simulink model "ADRConSiaAUV_ex02"  (R2021a)
settings: Solver=ode1  StartTime=0  StopTime=100  FixedStep=h  MaxStep=0.05  MinStep=0.005  RelTol=0.01
values from neighbouring files (symbols this model uses):
  b0 = 0.06    [tuning0325.m]
  h0 = 1.0    (= 1)    [tuning0325.m]
  kd = 10    [NPS_RBFNN01.m]    (also in SiaAUV_RBFNN01.m; SiaAUV_RBFNN02.m; SiaAUV_RBFNN03.m; tuning0325.m = 90)
  ki = 0.9    [tuning0325.m]
  kp = 6    [NPS_RBFNN01.m]    (also in SiaAUV_RBFNN01.m; SiaAUV_RBFNN02.m; SiaAUV_RBFNN03.m; tuning0325.m = 50)
  r0 = 0.8    [tuning0325.m]
  w0 = 80    [tuning0325.m]
  wc = 0.5    [tuning0325.m]
libraries: mssSimulink x12, simulink x3
settings Model: Creator=thor  LastModifiedBy=owenga
settings SolverCC: InitialStep=0.01  AlgebraicLoopSolver=TrustRegion  AutoInsertRateTranBlk=on
settings DataIOCC: LimitDataPoints=on  SaveFormat=Array  SignalLoggingSaveFormat=ModelDataLogs  ReturnWorkspaceOutputs=off  SignalLoggingName=sigsOut
settings OptimizationCC: BooleanDataType=off  InitFltsAndDblsToZero=on  LifeSpan=inf
settings DebuggingCC: SaveWithParameterizedLinksMsg=none  UnderspecifiedInitializationDetection=Classic  MergeDetectMultiDrivingBlocksExec=none  SignalResolutionControl=TryResolveAllWithWarning  MultiTaskDSMMsg=warning  MultiTaskCondExecSysMsg=none  FcnCallInpInsideContextMsg=warning  SFUnexpectedBacktrackingDiag=warning  SFNoUnconditionalDefaultTransitionDiag=warning  SFExecutionAtInitializationDiag=none  SFMachineParentedDataDiag=warning  ArithmeticOperatorsInVariantConditions=warning
settings HardwareCC: ProdBitPerPointer=32  ProdBitPerSizeT=32  ProdBitPerPtrDiffT=32  ProdLargestAtomicFloat=None  ProdIntDivRoundTo=Undefined  ProdEndianess=Unspecified  ProdWordSize=32  ProdHWDeviceType=32-bit Generic  TargetUnknown=on
settings ModelReferenceCC: PropagateSignalLabelsOutOfModel=off
settings CodeAppCC: StateflowObjectComments=on
settings GRTTargetCC: TargetFcnLib=ansi_tfl_tmw.mat  TargetLangStandard=C89/C90 (ANSI)  ModelReferenceCompliant=off  CombineOutputUpdateFcns=off  MatFileLogging=off  GRTInterface=on
settings ConfigComp: CovMetricSettings=dw  CovSaveCumulativeToWorkspaceVar=on  CovSaveSingleToWorkspaceVar=on

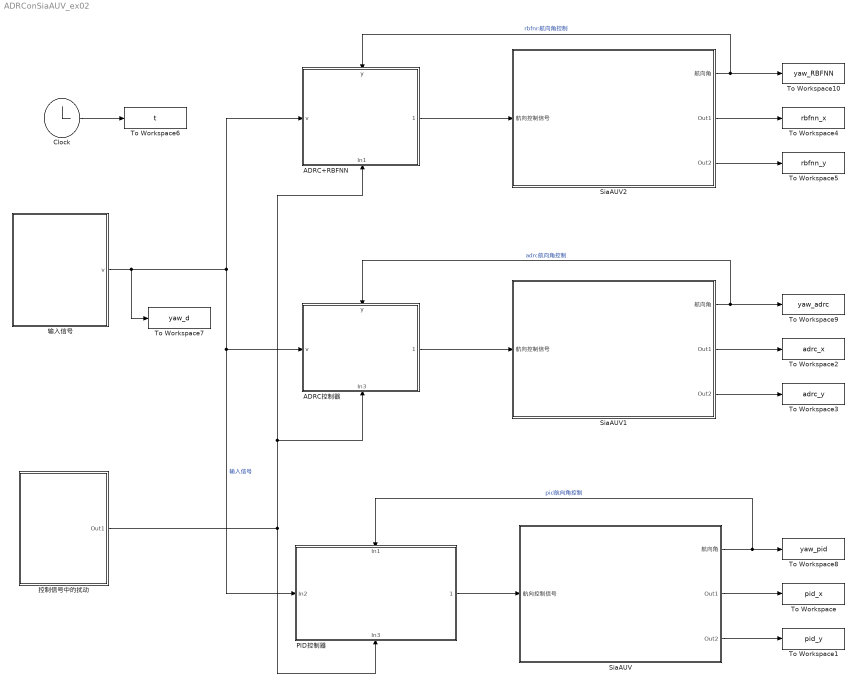
== system ADRConSiaAUV_ex02 ==
  ADRC+RBFNN : Subsystem
      settings: PortSchema="{\"entries\":[{\"content\":{\"sides\":[{\"content\":{\"connectorIds\":[\"In1\"]},\"type\":\"ConnectorPlacement.EquallySpacedRectSide\",\"uuid\":\"900b6237-364a-4e14-939f-8bb5c6ed2e80\"},{\"content\":{\"connectorIds\":[\"Out1\"],\"side\":\"RIGHT\"},\"type\":\"ConnectorPlacement.EquallySpacedRectSide\",\"uuid\":\"a73f2338-5f87-4ee3-a03f-e680a590baff\"},{\"content\":{\"connectorIds\":[\"In2\"],\"side\":\"TOP\"},\"type\":\"ConnectorPlacement.EquallySpacedRectSide\",\"uuid\":\"06c6f34a-b3b2-48d7-b766-545f9568804e\"},{\"content\":{\"connectorIds\":[\"In3\"],\"side\":\"BOTTOM\"},\"type\":\"ConnectorPlacement.EquallySpacedRectSide\",\"uuid\":\"dbaae600-9c02-41f2-84b1-a2698d1307a6\"}]},\"type\":\"ConnectorPlacement.EquallySpacedConnector\",\"uuid\":\"fa40750b-3e1f-406a-9fab-e6d49e04910d\"}],\"packageUris\":[\"http://schema.mathworks.com/mf0/Connector/R2020b\"],\"version\":\"1.0\"}"
  ADRC控制器 : Subsystem
      settings: PortSchema="{\"entries\":[{\"content\":{\"sides\":[{\"content\":{\"connectorIds\":[\"In1\"]},\"type\":\"ConnectorPlacement.EquallySpacedRectSide\",\"uuid\":\"32724ae5-2155-4067-bb70-245a7591a597\"},{\"content\":{\"connectorIds\":[\"Out1\"],\"side\":\"RIGHT\"},\"type\":\"ConnectorPlacement.EquallySpacedRectSide\",\"uuid\":\"c5581aa9-8b72-4f1c-be64-cbd035fc9c4e\"},{\"content\":{\"connectorIds\":[\"In2\"],\"side\":\"TOP\"},\"type\":\"ConnectorPlacement.EquallySpacedRectSide\",\"uuid\":\"d8180c3e-1afe-4e75-b9a0-261cdd740691\"},{\"content\":{\"connectorIds\":[\"In3\"],\"side\":\"BOTTOM\"},\"type\":\"ConnectorPlacement.EquallySpacedRectSide\",\"uuid\":\"8af971cc-81cd-4e66-97aa-994f656c03e7\"}]},\"type\":\"ConnectorPlacement.EquallySpacedConnector\",\"uuid\":\"6b6572c2-6358-4ebe-8c55-bca9fb0d42f3\"}],\"packageUris\":[\"http://schema.mathworks.com/mf0/Connector/R2020b\"],\"version\":\"1.0\"}"
  Clock : Clock
  PID控制器 : Subsystem
      settings: PortSchema="{\"entries\":[{\"content\":{\"sides\":[{\"content\":{\"connectorIds\":[\"In1\"]},\"type\":\"ConnectorPlacement.EquallySpacedRectSide\",\"uuid\":\"32724ae5-2155-4067-bb70-245a7591a597\"},{\"content\":{\"connectorIds\":[\"Out1\"],\"side\":\"RIGHT\"},\"type\":\"ConnectorPlacement.EquallySpacedRectSide\",\"uuid\":\"c5581aa9-8b72-4f1c-be64-cbd035fc9c4e\"},{\"content\":{\"connectorIds\":[\"In2\"],\"side\":\"TOP\"},\"type\":\"ConnectorPlacement.EquallySpacedRectSide\",\"uuid\":\"d8180c3e-1afe-4e75-b9a0-261cdd740691\"},{\"content\":{\"connectorIds\":[\"In3\"],\"side\":\"BOTTOM\"},\"type\":\"ConnectorPlacement.EquallySpacedRectSide\",\"uuid\":\"f6cb4f31-ad77-48c7-baef-a98beb6e51e5\"}]},\"type\":\"ConnectorPlacement.EquallySpacedConnector\",\"uuid\":\"6b6572c2-6358-4ebe-8c55-bca9fb0d42f3\"}],\"packageUris\":[\"http://schema.mathworks.com/mf0/Connector/R2020b\"],\"version\":\"1.0\"}"
  SiaAUV : Subsystem
  SiaAUV1 : Subsystem
  SiaAUV2 : Subsystem
  To Workspace : ToWorkspace  VariableName=pid_x  SampleTime=-1
  To Workspace1 : ToWorkspace  VariableName=pid_y  SampleTime=-1
  To Workspace10 : ToWorkspace  VariableName=yaw_RBFNN  SampleTime=-1
  To Workspace2 : ToWorkspace  VariableName=adrc_x  SampleTime=-1
  To Workspace3 : ToWorkspace  VariableName=adrc_y  SampleTime=-1
  To Workspace4 : ToWorkspace  VariableName=rbfnn_x  SampleTime=-1
  To Workspace5 : ToWorkspace  VariableName=rbfnn_y  SampleTime=-1
  To Workspace6 : ToWorkspace  VariableName=t  SampleTime=-1
  To Workspace7 : ToWorkspace  VariableName=yaw_d  SampleTime=-1
  To Workspace8 : ToWorkspace  VariableName=yaw_pid  SampleTime=-1
  To Workspace9 : ToWorkspace  VariableName=yaw_adrc  SampleTime=-1
  控制信号中的扰动 : Subsystem
  输入信号 : Subsystem
  wires:
  控制信号中的扰动/1(Out1) -> ADRC控制器/3(In3), ADRC+RBFNN/3(In1), PID控制器/3(In3)
  SiaAUV/1(航向角) -> PID控制器/2(In1), To Workspace8/1  "pid航向角控制"
  SiaAUV/2(Out1) -> To Workspace/1
  SiaAUV/3(Out2) -> To Workspace1/1
  输入信号/1(v) -> ADRC+RBFNN/1(v), PID控制器/1(In2), ADRC控制器/1(v), To Workspace7/1  "输入信号"
  ADRC控制器/1(1) -> SiaAUV1/1(航向控制信号)
  SiaAUV1/2(Out1) -> To Workspace2/1
  SiaAUV1/3(Out2) -> To Workspace3/1
  SiaAUV1/1(航向角) -> To Workspace9/1, ADRC控制器/2(y)  "adrc航向角控制"
  ADRC+RBFNN/1(1) -> SiaAUV2/1(航向控制信号)
  SiaAUV2/1(航向角) -> To Workspace10/1, ADRC+RBFNN/2(y)  "rbfnn航向角控制"
  SiaAUV2/2(Out1) -> To Workspace4/1
  SiaAUV2/3(Out2) -> To Workspace5/1
  PID控制器/1(1) -> SiaAUV/1(航向控制信号)
  Clock/1 -> To Workspace6/1

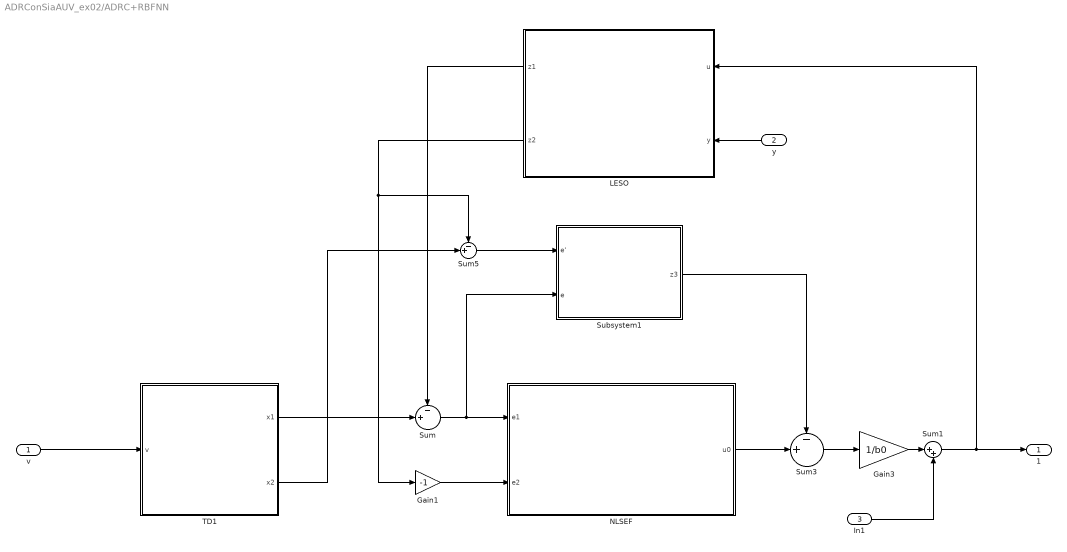
== system ADRConSiaAUV_ex02/ADRC+RBFNN ==
  v : Inport
  y : Inport  Port=2
  In1 : Inport  Port=3
  Gain1 : Gain  Gain=-1
  Gain3 : Gain  Gain=1/b0
  LESO : Subsystem
  NLSEF : Subsystem
  Subsystem1 : Subsystem
  Sum : Sum  Inputs=-+|
  Sum1 : Sum  Inputs=|++
  Sum3 : Sum  Inputs=-+|
  Sum5 : Sum  Inputs=-+|  SaturateOnIntegerOverflow=on
  TD1 : Subsystem
  1 : Outport
  wires:
  LESO/1(z1) -> Sum/1
  TD1/2(x2) -> Sum5/2
  NLSEF/1(u0) -> Sum3/2
  Sum5/1 -> Subsystem1/1(e')
  Sum3/1 -> Gain3/1
  Gain1/1 -> NLSEF/2(e2)
  y/1 -> LESO/2(y)
  Sum1/1 -> 1/1, LESO/1(u)
  LESO/2(z2) -> Gain1/1, Sum5/1
  Subsystem1/1(z3) -> Sum3/1
  Sum/1 -> Subsystem1/2(e), NLSEF/1(e1)
  Gain3/1 -> Sum1/1
  In1/1 -> Sum1/2
  v/1 -> TD1/1(v)
  TD1/1(x1) -> Sum/2

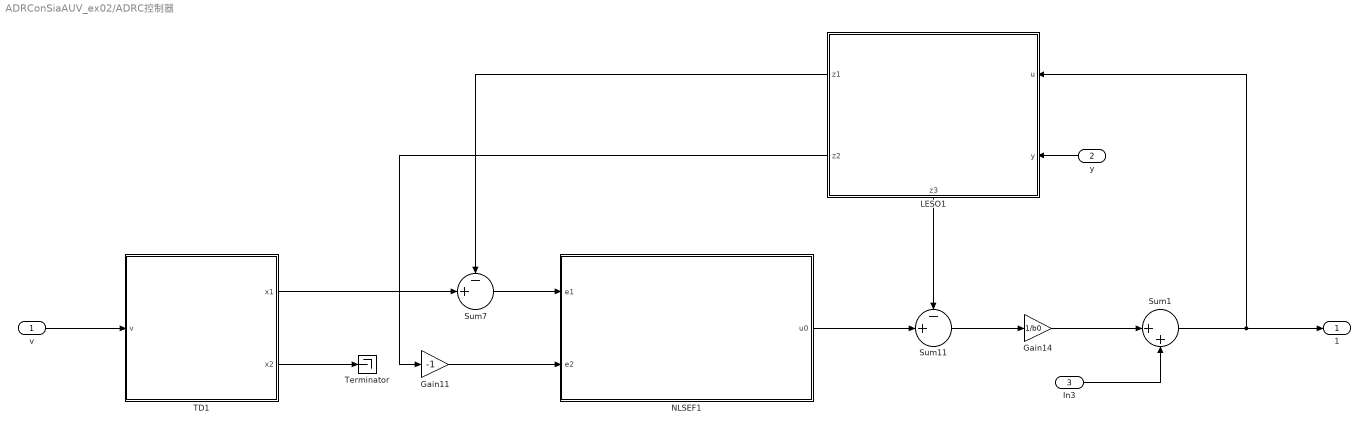
== system ADRConSiaAUV_ex02/ADRC控制器 ==
  v : Inport
  y : Inport  Port=2
  In3 : Inport  Port=3
  Gain11 : Gain  Gain=-1
  Gain14 : Gain  Gain=1/b0
  LESO1 : Subsystem
      settings: PortSchema="{\"entries\":[{\"content\":{\"sides\":[{\"content\":{\"connectorIds\":[\"In1\",\"In2\"]},\"type\":\"ConnectorPlacement.EquallySpacedRectSide\",\"uuid\":\"d43d14c0-31a6-421f-9c22-52af5a429c00\"},{\"content\":{\"connectorIds\":[\"Out1\",\"Out2\"],\"side\":\"RIGHT\"},\"type\":\"ConnectorPlacement.EquallySpacedRectSide\",\"uuid\":\"46ebe2a2-48dd-422a-a4e2-a7c2a0b0d12b\"},{\"content\":{\"connectorIds\":[],\"side\":\"TOP\"},\"type\":\"ConnectorPlacement.EquallySpacedRectSide\",\"uuid\":\"15fa3bf3-1107-4b09-8c97-c0a9c58ebc3c\"},{\"content\":{\"connectorIds\":[\"Out3\"],\"side\":\"BOTTOM\"},\"type\":\"ConnectorPlacement.EquallySpacedRectSide\",\"uuid\":\"1b52abbe-f0a6-429e-b5ef-1092e11e8dfa\"}]},\"type\":\"ConnectorPlacement.EquallySpacedConnector\",\"uuid\":\"aa00def6-f836-4863-9222-5c98f4f3fade\"}],\"packageUris\":[\"http://schema.mathworks.com/mf0/Connector/R2020b\"],\"version\":\"1.0\"}"
  NLSEF1 : Subsystem
  Sum1 : Sum  Inputs=|++
  Sum11 : Sum  Inputs=-+|
  Sum7 : Sum  Inputs=-+|
  TD1 : Subsystem
  Terminator : Terminator
  1 : Outport
  wires:
  LESO1/1(z1) -> Sum7/1
  Sum11/1 -> Gain14/1
  Gain11/1 -> NLSEF1/2(e2)
  TD1/1(x1) -> Sum7/2
  NLSEF1/1(u0) -> Sum11/2
  y/1 -> LESO1/2(y)
  Sum1/1 -> LESO1/1(u), 1/1
  TD1/2(x2) -> Terminator/1
  LESO1/2(z2) -> Gain11/1
  In3/1 -> Sum1/2
  Gain14/1 -> Sum1/1
  LESO1/3(z3) -> Sum11/1
  v/1 -> TD1/1(v)
  Sum7/1 -> NLSEF1/1(e1)

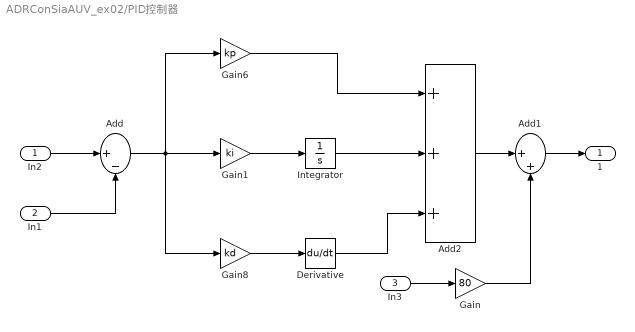
== system ADRConSiaAUV_ex02/PID控制器 ==
  In2 : Inport
  In1 : Inport  Port=2
  In3 : Inport  Port=3
  Add : Sum  Inputs=|+-
  Add1 : Sum  Inputs=|++
  Add2 : Sum  Inputs=+++
  Derivative : Derivative
  Gain : Gain  Gain=80
  Gain1 : Gain  Gain=ki
  Gain6 : Gain  Gain=kp
  Gain8 : Gain  Gain=kd
  Integrator : Integrator
  1 : Outport
  wires:
  In1/1 -> Add/2
  Add1/1 -> 1/1
  In2/1 -> Add/1
  In3/1 -> Gain/1
  Add2/1 -> Add1/1
  Derivative/1 -> Add2/3
  Gain8/1 -> Derivative/1
  Gain1/1 -> Integrator/1
  Integrator/1 -> Add2/2
  Gain6/1 -> Add2/1
  Add/1 -> Gain1/1, Gain8/1, Gain6/1
  Gain/1 -> Add1/2

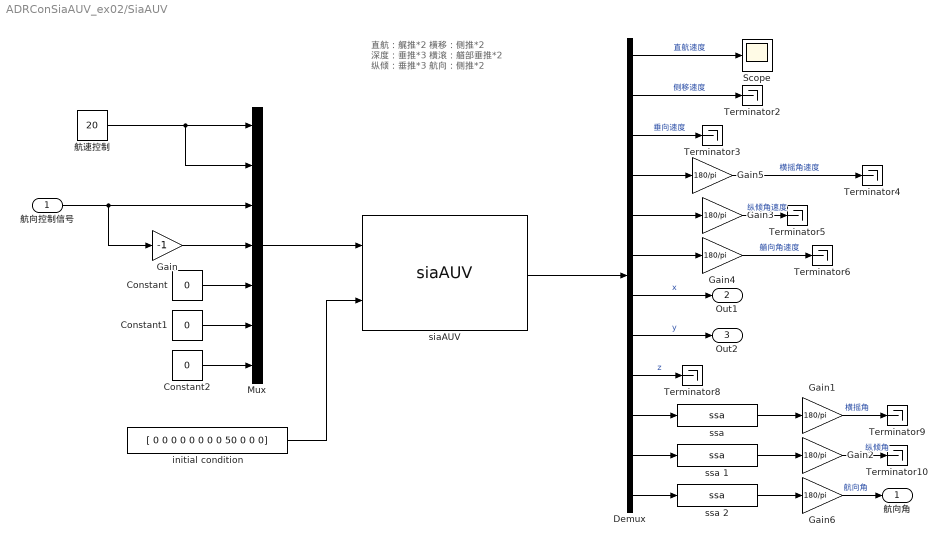
== system ADRConSiaAUV_ex02/SiaAUV ==
  note: 直航：艉推*2
      | 横移：侧推*2
      | 深度：垂推*3
      | 横滚：艏部垂推*2
      | 纵倾：垂推*3
      | 航向：侧推*2
  航向控制信号 : Inport
  Constant : Constant  Value=0
  Constant1 : Constant  Value=0
  Constant2 : Constant  Value=0
  Demux : Demux  Outputs=12
  Gain : Gain  Gain=-1
  Gain{1..6} (6 alike) : Gain  Gain=180/pi
  Mux : Mux  Inputs=[1 1 1 1 1 1 1]
  Scope : Scope
  Terminator{2..6,8..10} (8 alike) : Terminator
  initial condition : Constant  Value=[ 0 0 0 0 0 0 0 0 50 0 0 0]
  siaAUV : mssSimulink/Marine craft models/siaAUV  SystemSampleTime=-1  VariantActivationTime=update diagram  Latency=0  AutoFrameSizeCalculation=off
      settings: SourceProductName=Under Water Robot Toolbox
  "ssa " : mssSimulink/Utilities/Math Operations/ssa  SystemSampleTime=-1  VariantActivationTime=update diagram  Latency=0  AutoFrameSizeCalculation=off
      settings: SourceProductName=Under Water Robot Toolbox
  ssa 1 : mssSimulink/Utilities/Math Operations/ssa  SystemSampleTime=-1  VariantActivationTime=update diagram  Latency=0  AutoFrameSizeCalculation=off
      settings: SourceProductName=Under Water Robot Toolbox
  ssa 2 : mssSimulink/Utilities/Math Operations/ssa  SystemSampleTime=-1  VariantActivationTime=update diagram  Latency=0  AutoFrameSizeCalculation=off
      settings: SourceProductName=Under Water Robot Toolbox
  航速控制 : Constant  Value=20
  航向角 : Outport
  Out1 : Outport  Port=2
  Out2 : Outport  Port=3
  wires:
  Gain3/1 -> Terminator5/1  "纵倾角速度"
  Demux/3 -> Terminator3/1  "垂向速度"
  Gain1/1 -> Terminator9/1  "横摇角"
  Demux/4 -> Gain5/1
  Constant/1 -> Mux/5
  Gain/1 -> Mux/4
  Demux/12 -> ssa 2/1
  siaAUV/1 -> Demux/1
  ssa 1/1 -> Gain2/1
  Demux/5 -> Gain3/1
  Demux/9 -> Terminator8/1  "z"
  Demux/7 -> Out1/1  "x"
  Constant2/1 -> Mux/7
  ssa 2/1 -> Gain6/1
  Demux/1 -> Scope/1  "直航速度"
  Gain4/1 -> Terminator6/1  "艏向角速度"
  Demux/10 -> "ssa "/1
  Constant1/1 -> Mux/6
  initial condition/1 -> siaAUV/2
  "ssa "/1 -> Gain1/1
  Demux/6 -> Gain4/1
  Gain2/1 -> Terminator10/1  "纵倾角"
  Gain5/1 -> Terminator4/1  "横摇角速度"
  航速控制/1 -> Mux/2, Mux/1
  Demux/11 -> ssa 1/1
  Demux/2 -> Terminator2/1  "侧移速度"
  Gain6/1 -> 航向角/1  "航向角"
  Mux/1 -> siaAUV/1
  Demux/8 -> Out2/1  "y"
  航向控制信号/1 -> Gain/1, Mux/3

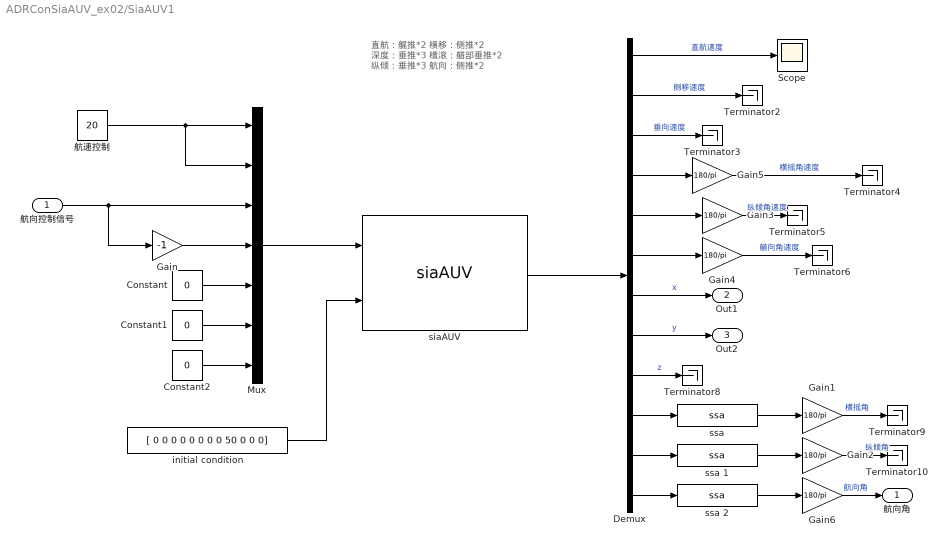
== system ADRConSiaAUV_ex02/SiaAUV1 ==
  note: 直航：艉推*2
      | 横移：侧推*2
      | 深度：垂推*3
      | 横滚：艏部垂推*2
      | 纵倾：垂推*3
      | 航向：侧推*2
  航向控制信号 : Inport
  Constant : Constant  Value=0
  Constant1 : Constant  Value=0
  Constant2 : Constant  Value=0
  Demux : Demux  Outputs=12
  Gain : Gain  Gain=-1
  Gain{1..6} (6 alike) : Gain  Gain=180/pi
  Mux : Mux  Inputs=[1 1 1 1 1 1 1]
  Scope : Scope
  Terminator{2..6,8..10} (8 alike) : Terminator
  initial condition : Constant  Value=[ 0 0 0 0 0 0 0 0 50 0 0 0]
  siaAUV : mssSimulink/Marine craft models/siaAUV  SystemSampleTime=-1  VariantActivationTime=update diagram  Latency=0  AutoFrameSizeCalculation=off
      settings: SourceProductName=Under Water Robot Toolbox
  "ssa " : mssSimulink/Utilities/Math Operations/ssa  SystemSampleTime=-1  VariantActivationTime=update diagram  Latency=0  AutoFrameSizeCalculation=off
      settings: SourceProductName=Under Water Robot Toolbox
  ssa 1 : mssSimulink/Utilities/Math Operations/ssa  SystemSampleTime=-1  VariantActivationTime=update diagram  Latency=0  AutoFrameSizeCalculation=off
      settings: SourceProductName=Under Water Robot Toolbox
  ssa 2 : mssSimulink/Utilities/Math Operations/ssa  SystemSampleTime=-1  VariantActivationTime=update diagram  Latency=0  AutoFrameSizeCalculation=off
      settings: SourceProductName=Under Water Robot Toolbox
  航速控制 : Constant  Value=20
  航向角 : Outport
  Out1 : Outport  Port=2
  Out2 : Outport  Port=3
  wires:
  航向控制信号/1 -> Mux/3, Gain/1
  Demux/8 -> Out2/1  "y"
  Mux/1 -> siaAUV/1
  Gain6/1 -> 航向角/1  "航向角"
  Demux/2 -> Terminator2/1  "侧移速度"
  Demux/11 -> ssa 1/1
  航速控制/1 -> Mux/1, Mux/2
  Gain5/1 -> Terminator4/1  "横摇角速度"
  Gain2/1 -> Terminator10/1  "纵倾角"
  Demux/6 -> Gain4/1
  "ssa "/1 -> Gain1/1
  initial condition/1 -> siaAUV/2
  Constant1/1 -> Mux/6
  Demux/10 -> "ssa "/1
  Gain4/1 -> Terminator6/1  "艏向角速度"
  Demux/1 -> Scope/1  "直航速度"
  ssa 2/1 -> Gain6/1
  Constant2/1 -> Mux/7
  Demux/7 -> Out1/1  "x"
  Demux/9 -> Terminator8/1  "z"
  Demux/5 -> Gain3/1
  ssa 1/1 -> Gain2/1
  siaAUV/1 -> Demux/1
  Demux/12 -> ssa 2/1
  Gain/1 -> Mux/4
  Constant/1 -> Mux/5
  Demux/4 -> Gain5/1
  Gain1/1 -> Terminator9/1  "横摇角"
  Demux/3 -> Terminator3/1  "垂向速度"
  Gain3/1 -> Terminator5/1  "纵倾角速度"

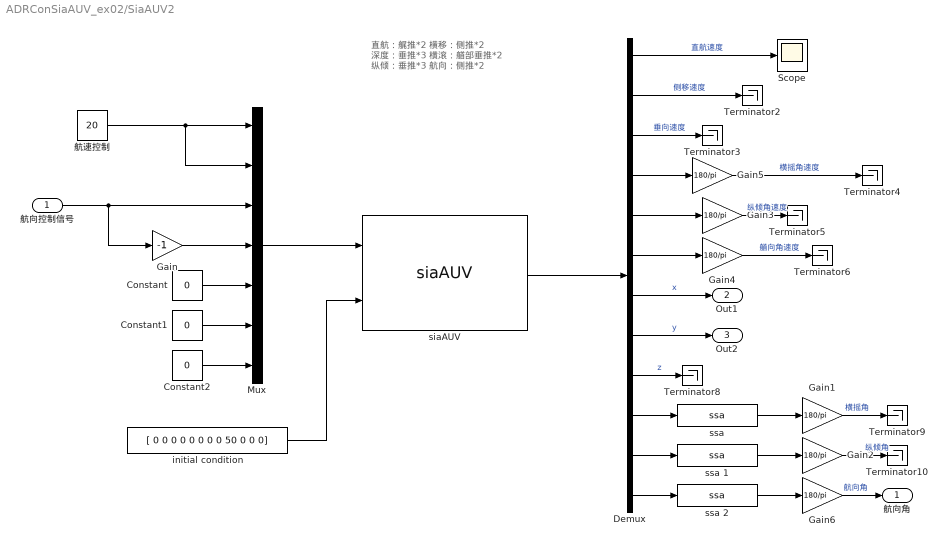
== system ADRConSiaAUV_ex02/SiaAUV2 ==
  note: 直航：艉推*2
      | 横移：侧推*2
      | 深度：垂推*3
      | 横滚：艏部垂推*2
      | 纵倾：垂推*3
      | 航向：侧推*2
  航向控制信号 : Inport
  Constant : Constant  Value=0
  Constant1 : Constant  Value=0
  Constant2 : Constant  Value=0
  Demux : Demux  Outputs=12
  Gain : Gain  Gain=-1
  Gain{1..6} (6 alike) : Gain  Gain=180/pi
  Mux : Mux  Inputs=[1 1 1 1 1 1 1]
  Scope : Scope
  Terminator{2..6,8..10} (8 alike) : Terminator
  initial condition : Constant  Value=[ 0 0 0 0 0 0 0 0 50 0 0 0]
  siaAUV : mssSimulink/Marine craft models/siaAUV  SystemSampleTime=-1  VariantActivationTime=update diagram  Latency=0  AutoFrameSizeCalculation=off
      settings: SourceProductName=Under Water Robot Toolbox
  "ssa " : mssSimulink/Utilities/Math Operations/ssa  SystemSampleTime=-1  VariantActivationTime=update diagram  Latency=0  AutoFrameSizeCalculation=off
      settings: SourceProductName=Under Water Robot Toolbox
  ssa 1 : mssSimulink/Utilities/Math Operations/ssa  SystemSampleTime=-1  VariantActivationTime=update diagram  Latency=0  AutoFrameSizeCalculation=off
      settings: SourceProductName=Under Water Robot Toolbox
  ssa 2 : mssSimulink/Utilities/Math Operations/ssa  SystemSampleTime=-1  VariantActivationTime=update diagram  Latency=0  AutoFrameSizeCalculation=off
      settings: SourceProductName=Under Water Robot Toolbox
  航速控制 : Constant  Value=20
  航向角 : Outport
  Out1 : Outport  Port=2
  Out2 : Outport  Port=3
  wires:
  Gain3/1 -> Terminator5/1  "纵倾角速度"
  Demux/3 -> Terminator3/1  "垂向速度"
  Gain1/1 -> Terminator9/1  "横摇角"
  Demux/4 -> Gain5/1
  Constant/1 -> Mux/5
  Gain/1 -> Mux/4
  Demux/12 -> ssa 2/1
  siaAUV/1 -> Demux/1
  ssa 1/1 -> Gain2/1
  Demux/5 -> Gain3/1
  Demux/9 -> Terminator8/1  "z"
  Demux/7 -> Out1/1  "x"
  Constant2/1 -> Mux/7
  ssa 2/1 -> Gain6/1
  Demux/1 -> Scope/1  "直航速度"
  Gain4/1 -> Terminator6/1  "艏向角速度"
  Demux/10 -> "ssa "/1
  Constant1/1 -> Mux/6
  initial condition/1 -> siaAUV/2
  "ssa "/1 -> Gain1/1
  Demux/6 -> Gain4/1
  Gain2/1 -> Terminator10/1  "纵倾角"
  Gain5/1 -> Terminator4/1  "横摇角速度"
  航速控制/1 -> Mux/2, Mux/1
  Demux/11 -> ssa 1/1
  Demux/2 -> Terminator2/1  "侧移速度"
  Gain6/1 -> 航向角/1  "航向角"
  Mux/1 -> siaAUV/1
  Demux/8 -> Out2/1  "y"
  航向控制信号/1 -> Gain/1, Mux/3

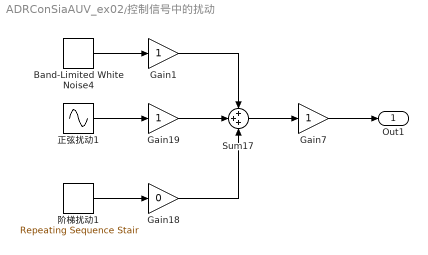
== system ADRConSiaAUV_ex02/控制信号中的扰动 ==
  Band-Limited White Noise4 : simulink/Sources/Band-Limited White Noise  Cov=[0.0005]  Ts=0.01  seed=[23341]
  Gain1 : Gain
  Gain18 : Gain  Gain=0
  Gain19 : Gain
  Gain7 : Gain
  Sum17 : Sum  Inputs=+++
  正弦扰动1 : Sin  Amplitude=2  Frequency=0.1*pi  SampleTime=0
  阶梯扰动1 : simulink/Sources/Repeating Sequence Stair  OutValues=[1 -1].'  tsamp=5  OutMin=[]  OutMax=[]  OutDataTypeStr=double  OutputDataTypeScalingMode=double  OutDataType=fixdt(0,8)  ConRadixGroup=Best Precision: Vector-wise  OutScaling=2^-12
  Out1 : Outport
  wires:
  Gain7/1 -> Out1/1
  Sum17/1 -> Gain7/1
  Gain18/1 -> Sum17/3
  Gain19/1 -> Sum17/2
  正弦扰动1/1 -> Gain19/1
  阶梯扰动1/1 -> Gain18/1
  Band-Limited White Noise4/1 -> Gain1/1
  Gain1/1 -> Sum17/1

== system ADRConSiaAUV_ex02/输入信号 ==
  Gain : Gain  Gain=0
  Gain1 : Gain
  Repeating Sequence Stair : simulink/Sources/Repeating Sequence Stair  OutValues=[10 -10].'  tsamp=30  OutMin=[]  OutMax=[]  OutDataTypeStr=double  OutputDataTypeScalingMode=double  OutDataType=fixdt(0,8)  ConRadixGroup=Best Precision: Vector-wise  OutScaling=2^-12
  Step : Step  Time=10  After=10  SampleTime=0
  Sum : Sum  Inputs=++|
  Transport Delay : TransportDelay  DelayTime=10  BufferSize=2048
  v : Outport
  wires:
  Sum/1 -> v/1
  Repeating Sequence Stair/1 -> Transport Delay/1
  Step/1 -> Gain/1
  Gain/1 -> Sum/1
  Gain1/1 -> Sum/2
  Transport Delay/1 -> Gain1/1

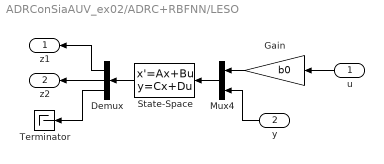
== system ADRConSiaAUV_ex02/ADRC+RBFNN/LESO ==
  u : Inport
  y : Inport  Port=2
  Demux : Demux  Outputs=3
  Gain : Gain  Gain=b0
  Mux4 : Mux  Inputs=2
  State-Space : StateSpace  A=[-3*w0 1 0; -3*w0^2 0 1; -w0^3 0 0]  B=[0 3*w0; 1 3*w0^2; 0 w0^3]  C=[1 0 0; 0 1 0; 0 0 1]  D=[0 0; 0 0; 0 0]  InitialCondition=0
  Terminator : Terminator
  z1 : Outport
  z2 : Outport  Port=2
  wires:
  Demux/1 -> z1/1
  u/1 -> Gain/1
  y/1 -> Mux4/2
  Mux4/1 -> State-Space/1
  Demux/2 -> z2/1
  State-Space/1 -> Demux/1
  Demux/3 -> Terminator/1
  Gain/1 -> Mux4/1

== system ADRConSiaAUV_ex02/ADRC+RBFNN/NLSEF ==
  e1 : Inport
  e2 : Inport  Port=2
  Add : Sum
  kd : Gain  Gain=2*wc
  kp : Gain  Gain=wc^2
  u0 : Outport
  wires:
  e1/1 -> kp/1
  e2/1 -> kd/1
  Add/1 -> u0/1
  kp/1 -> Add/1
  kd/1 -> Add/2

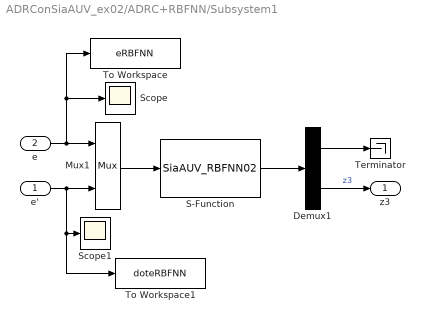
== system ADRConSiaAUV_ex02/ADRC+RBFNN/Subsystem1 ==
  e' : Inport
  e : Inport  Port=2
  Demux1 : Demux  Outputs=2
      settings: DisplayOption=none
  Mux1 : Mux  Inputs=2
  S-Function : S-Function  FunctionName=SiaAUV_RBFNN02  SFunctionDeploymentMode=off  EnableBusSupport=off
  Scope : Scope
  Scope1 : Scope
  Terminator : Terminator
  To Workspace : ToWorkspace  VariableName=eRBFNN  SaveFormat=Structure With Time  SampleTime=-1
  To Workspace1 : ToWorkspace  VariableName=doteRBFNN  SaveFormat=Structure With Time  SampleTime=-1
  z3 : Outport
  wires:
  e/1 -> To Workspace/1, Scope/1, Mux1/1
  Demux1/2 -> z3/1  "z3"
  S-Function/1 -> Demux1/1
  e'/1 -> To Workspace1/1, Scope1/1, Mux1/2
  Demux1/1 -> Terminator/1
  Mux1/1 -> S-Function/1

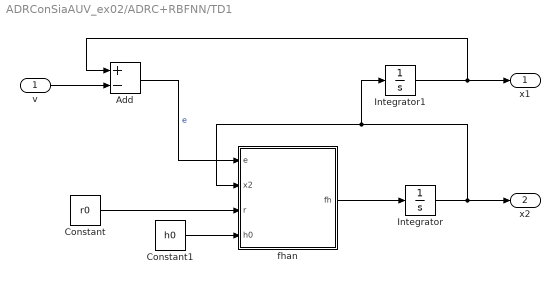
== system ADRConSiaAUV_ex02/ADRC+RBFNN/TD1 ==
  v : Inport
  Add : Sum  Inputs=+-
  Constant : Constant  Value=r0
  Constant1 : Constant  Value=h0
  Integrator : Integrator
  Integrator1 : Integrator
  fhan : MATLAB Function  TreatAsAtomicUnit=on
  x1 : Outport
  x2 : Outport  Port=2
  wires:
  v/1 -> Add/2
  Integrator1/1 -> Add/1, x1/1
  Add/1 -> fhan/1(e)  "e"
  fhan/1(fh) -> Integrator/1
  Integrator/1 -> x2/1, Integrator1/1, fhan/2(x2)
  Constant/1 -> fhan/3(r)
  Constant1/1 -> fhan/4(h0)

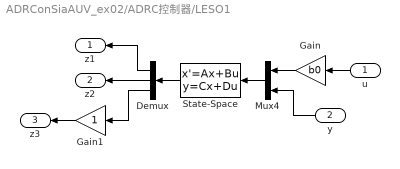
== system ADRConSiaAUV_ex02/ADRC控制器/LESO1 ==
  u : Inport
  y : Inport  Port=2
  Demux : Demux  Outputs=3
  Gain : Gain  Gain=b0
  Gain1 : Gain
  Mux4 : Mux  Inputs=2
  State-Space : StateSpace  A=[-3*w0 1 0; -3*w0^2 0 1; -w0^3 0 0]  B=[0 3*w0; 1 3*w0^2; 0 w0^3]  C=[1 0 0; 0 1 0; 0 0 1]  D=[0 0; 0 0; 0 0]  InitialCondition=0
  z1 : Outport
  z2 : Outport  Port=2
  z3 : Outport  Port=3
  wires:
  Demux/1 -> z1/1
  u/1 -> Gain/1
  y/1 -> Mux4/2
  Mux4/1 -> State-Space/1
  Demux/2 -> z2/1
  State-Space/1 -> Demux/1
  Demux/3 -> Gain1/1
  Gain/1 -> Mux4/1
  Gain1/1 -> z3/1

== system ADRConSiaAUV_ex02/ADRC控制器/NLSEF1 ==
  e1 : Inport
  e2 : Inport  Port=2
  Add : Sum
  kd : Gain  Gain=2*wc
  kp : Gain  Gain=wc^2
  u0 : Outport
  wires:
  e1/1 -> kp/1
  e2/1 -> kd/1
  Add/1 -> u0/1
  kp/1 -> Add/1
  kd/1 -> Add/2

== system ADRConSiaAUV_ex02/ADRC控制器/TD1 ==
  v : Inport
  Add : Sum  Inputs=+-
  Constant : Constant  Value=r0
  Constant1 : Constant  Value=h0
  Integrator : Integrator
  Integrator1 : Integrator
  fhan : MATLAB Function  TreatAsAtomicUnit=on
  x1 : Outport
  x2 : Outport  Port=2
  wires:
  v/1 -> Add/2
  Integrator1/1 -> Add/1, x1/1
  Add/1 -> fhan/1(e)  "e"
  fhan/1(fh) -> Integrator/1
  Integrator/1 -> x2/1, Integrator1/1, fhan/2(x2)
  Constant/1 -> fhan/3(r)
  Constant1/1 -> fhan/4(h0)

== matlab function ADRConSiaAUV_ex02/ADRC控制器/TD1/fhan ==
  data: e input; fh output; x2 input; r input; h0 input
function fh = fhan(e, x2, r, h0)
%最速跟踪微分器

d=r*h0^2;
a0=h0*x2;
y=e+a0;
a1=sqrt(d*(d+8*abs(y)));
a2=a0+sign(y)*(a1-d)/2;
a=(a0+y)*(sign(y+d)-sign(y-d))/2+a2*(1-(sign(y+d)-sign(y-d))/2);
fh = -r*(a/d)*(sign(a+d)-sign(a-d))/2-r*sign(a)*(1-(sign(a+d)-sign(a-d))/2);

== matlab function ADRConSiaAUV_ex02/ADRC+RBFNN/TD1/fhan ==
  data: e input; fh output; x2 input; r input; h0 input
function fh = fhan(e, x2, r, h0)
%最速跟踪微分器

d=r*h0^2;
a0=h0*x2;
y=e+a0;
a1=sqrt(d*(d+8*abs(y)));
a2=a0+sign(y)*(a1-d)/2;
a=(a0+y)*(sign(y+d)-sign(y-d))/2+a2*(1-(sign(y+d)-sign(y-d))/2);
fh = -r*(a/d)*(sign(a+d)-sign(a-d))/2-r*sign(a)*(1-(sign(a+d)-sign(a-d))/2);
